simulink model "HybridSystem"  (R2013a)
settings: Solver=ode45  StartTime=0.0  StopTime=75  RelTol=1e-3
undefined symbols (not defined in the file or in its folder): DiscIntNeverNeededParam
settings Model: Creator=Avisek Naug  LastModifiedBy=Avisek Naug

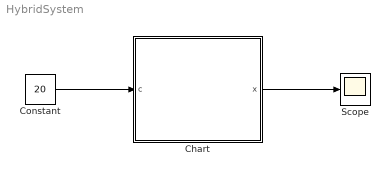
== system HybridSystem ==
  Chart : Stateflow chart  TreatAsAtomicUnit=on
  Constant : Constant  Value=20
  Scope : Scope
  wires:
  Constant/1 -> Chart/1(c)
  Chart/1(x) -> Scope/1

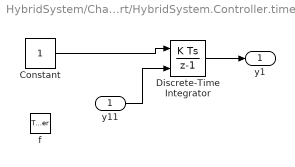
== system HybridSystem/Chart/HybridSystem.Controller.timer1 ==
  y11 : Inport
  f : TriggerPort  TriggerType=function-call
      settings: CopyFcn=Stateflow.SLINSF.SimulinkMan.removeBlockPreDeleteFcn  PreDeleteFcn=Stateflow.SLINSF.SimulinkMan.unsafePredeleteFcn
  Constant : Constant
  Discrete-Time Integrator : DiscreteIntegrator  InitialConditionSource=external  SampleTime=-1  ICPrevOutput=DiscIntNeverNeededParam  ICPrevScaledInput=DiscIntNeverNeededParam
  y1 : Outport
  wires:
  y11/1 -> Discrete-Time Integrator/2
  Constant/1 -> Discrete-Time Integrator/1
  Discrete-Time Integrator/1 -> y1/1

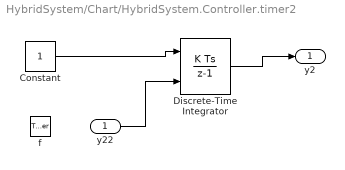
== system HybridSystem/Chart/HybridSystem.Controller.timer2 ==
  y22 : Inport
  f : TriggerPort  TriggerType=function-call
      settings: CopyFcn=Stateflow.SLINSF.SimulinkMan.removeBlockPreDeleteFcn  PreDeleteFcn=Stateflow.SLINSF.SimulinkMan.unsafePredeleteFcn
  Constant : Constant
  Discrete-Time Integrator : DiscreteIntegrator  InitialConditionSource=external  SampleTime=-1  ICPrevOutput=DiscIntNeverNeededParam  ICPrevScaledInput=DiscIntNeverNeededParam
  y2 : Outport
  wires:
  Discrete-Time Integrator/1 -> y2/1
  y22/1 -> Discrete-Time Integrator/2
  Constant/1 -> Discrete-Time Integrator/1

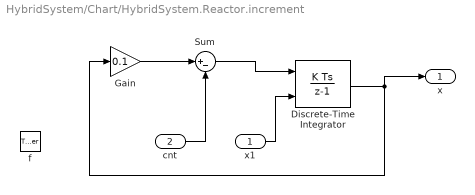
== system HybridSystem/Chart/HybridSystem.Reactor.increment ==
  x1 : Inport
  cnt : Inport  Port=2
  f : TriggerPort  TriggerType=function-call
      settings: CopyFcn=Stateflow.SLINSF.SimulinkMan.removeBlockPreDeleteFcn  PreDeleteFcn=Stateflow.SLINSF.SimulinkMan.unsafePredeleteFcn
  Discrete-Time Integrator : DiscreteIntegrator  InitialConditionSource=external  SampleTime=-1  ICPrevOutput=DiscIntNeverNeededParam  ICPrevScaledInput=DiscIntNeverNeededParam
  Gain : Gain  Gain=0.1
  Sum : Sum  Inputs=|+-
  x : Outport
  wires:
  Discrete-Time Integrator/1 -> x/1, Gain/1
  x1/1 -> Discrete-Time Integrator/2
  cnt/1 -> Sum/2
  Sum/1 -> Discrete-Time Integrator/1
  Gain/1 -> Sum/1

== stateflow chart HybridSystem/Chart ==
  state HybridSystem
    state Reactor [parallel]
      settings: executionOrder=1
      state Rod1
        en:
        x1 = x;
        cnt = 56;
        du:
        x = increment(x1,cnt);
      state NoRod
        en:
        x1 = x;
        cnt = 50;
        du:
        x = increment(x1,cnt);
      state Rod2
        en:
        x1 = x;
        cnt = 60;
        du:
        x = increment(x1,cnt);
      state x = increment(x1,cnt) [function]
      HybridSystem.Reactor.NoRod -> HybridSystem.Reactor.Rod1 [order 1] : add1
      (default) -> HybridSystem.Reactor.NoRod : {x = 510;}
      HybridSystem.Reactor.Rod1 -> HybridSystem.Reactor.NoRod : remove1
      HybridSystem.Reactor.Rod2 -> HybridSystem.Reactor.NoRod : remove2
      HybridSystem.Reactor.NoRod -> HybridSystem.Reactor.Rod2 [order 2] : add2
    state Controller [parallel]
      settings: executionOrder=2
      state Rod1
        en:
        y11 = y1;
        y22 = y2;
        du:
        y1 = timer1(y11);
        y2 = timer2(y22);
      state NoRod
        en:
        y11 = y1;
        y22 = y2;
        du:
        y1 = timer1(y11);
        y2 = timer2(y22);
      state Rod2
        en:
        y11 = y1;
        y22 = y2;
        du:
        y1 = timer1(y11);
        y2 = timer2(y22);
      state y1 = timer1(y11) [function]
      state y2 = timer2(y22) [function]
      HybridSystem.Controller.NoRod -> HybridSystem.Controller.Rod1 [order 1] : [x>=550&y1>=c&y2<c]/{send(add1)}
      (default) -> HybridSystem.Controller.NoRod : {y1 = c;
          | y2 = c;}
      HybridSystem.Controller.Rod1 -> HybridSystem.Controller.NoRod : [x<=510]/{send(remove1);y1 = 0;}
      HybridSystem.Controller.NoRod -> HybridSystem.Controller.Rod2 [order 2] : [x>=550&y2>=c]/{send(add2)}
      HybridSystem.Controller.Rod2 -> HybridSystem.Controller.NoRod : [x<=510]/{send(remove2);y2=0;}
  (default) -> HybridSystem
  data: x function_output; x1 function_input; cnt function_input; x1 local double; y11 function_input; y1 function_output; y22 function_input; y2 function_output; y1 local double; y11 local double; y2 local double; y22 local double; cnt local double; x output double; c input double
  events: add1 local FUNCTION_CALL_EVENT; add2 local FUNCTION_CALL_EVENT; remove1 local FUNCTION_CALL_EVENT; remove2 local FUNCTION_CALL_EVENT
